simulink model "Ball"  (Simulink 9.3)
settings: Solver=ode45  StartTime=0.0  StopTime=10.0  RelTol=1e-3  EnableMultiTasking=on
settings Model: Creator=baidx  LastModifiedBy=BEAR
settings DataIOCC: LimitDataPoints=on  SignalLoggingSaveFormat=Dataset
settings DebuggingCC: UnderspecifiedInitializationDetection=Simplified  MergeDetectMultiDrivingBlocksExec=error  SolverPrmCheckMsg=warning  FcnCallInpInsideContextMsg=error
settings GRTTargetCC: GeneratePreprocessorConditionals=Disable all  CombineOutputUpdateFcns=on  GRTInterface=off
settings ConfigComp: CovSFcnEnable=off

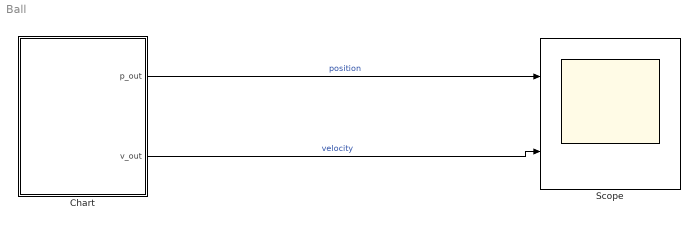
== system Ball ==
  Chart : Stateflow chart  TreatAsAtomicUnit=on
  Scope : Scope  NumInputPorts=2
  wires:
  Chart/1(p_out) -> Scope/1  "position"
  Chart/2(v_out) -> Scope/2  "velocity"

== stateflow chart Chart ==
  settings: updateMethod=CONTINUOUS
  state Falling
    during:
    p_dot=v;
    v_dot=-9.81;
    p_out=p;
    v_out=v;
  (default) -> Falling : {p=10;v=15}
  Falling -> Falling : [p<=0&&v<0]{p=0;v=-0.8*v}
  data: p_out output double; v_out output double; p local double; v local double
  data p settings: updateMethod=SF_CONTINUOUS_TIME_DATA
  data v settings: updateMethod=SF_CONTINUOUS_TIME_DATA
